simulink subsystem "Motor_Cmd"  (R2023b)
settings: Solver=VariableStepAuto  StartTime=0.0  StopTime=10.0  RelTol=1e-3
settings Model: Creator=m4ttn  LastModifiedBy=m4ttn

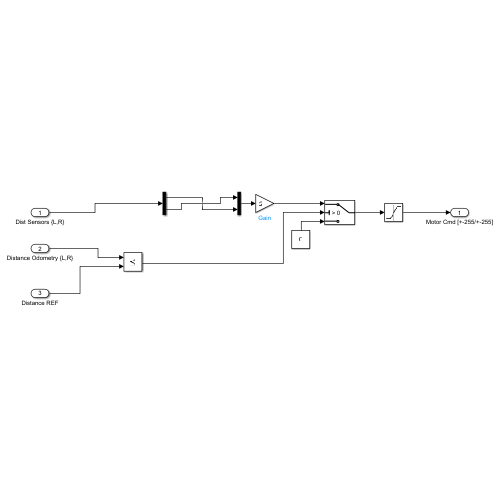
[thumbnail: Simulink's stored preview of the top-level diagram]
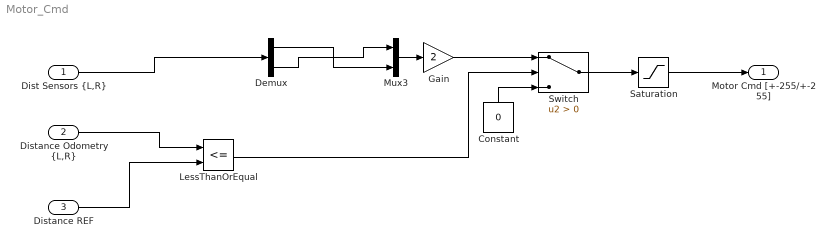
== system Motor_Cmd ==
  "Dist Sensors {L,R}" : Inport
  "Distance Odometry {L,R}" : Inport  Port=2
  Distance REF : Inport  Port=3
  Constant : Constant  Value=0  OutDataTypeStr=uint16
  Demux : Demux  Outputs=2
  Gain : Gain  Gain=2  ParamDataTypeStr=uint16  OutDataTypeStr=uint16
  LessThanOrEqual : RelationalOperator  Operator=<=  OutDataTypeStr=boolean  RndMeth=Simplest  InputSameDT=off
  Mux3 : Mux  Inputs=2
  Saturation : Saturate  UpperLimit=100  LowerLimit=0  OutDataTypeStr=int16
  Switch : Switch  Criteria=u2 > Threshold  SaturateOnIntegerOverflow=off  InputSameDT=off
  Motor Cmd [+-255/+-255] : Outport
  wires:
  Mux3/1 -> Gain/1
  Demux/2 -> Mux3/1
  "Dist Sensors {L,R}"/1 -> Demux/1
  Gain/1 -> Switch/1
  LessThanOrEqual/1 -> Switch/2
  Constant/1 -> Switch/3
  Switch/1 -> Saturation/1
  Saturation/1 -> Motor Cmd [+-255/+-255]/1
  "Distance Odometry {L,R}"/1 -> LessThanOrEqual/1
  Distance REF/1 -> LessThanOrEqual/2
  Demux/1 -> Mux3/2
